simulink model "uz_typeconv_27En18_to27En15"  (R2021a)
settings: Solver=FixedStepDiscrete  StartTime=0.0  StopTime=0.1  RelTol=1e-3
values from neighbouring files (symbols this model uses):
  t_ADC = 1/f_ADC    (= 1e-05)    [uz_6ph_pu_vsd_voltages_init.m]    (also in uz_mpc_6ph_init.m; uz_mpc_6ph_state_machine_init.m; uz_typeconv_init.m)
libraries: simulink x1
settings Model: DataTypeOverride=Off  Creator=micha  LastModifiedBy=micha
settings SolverCC: AlgebraicLoopSolver=TrustRegion
settings DataIOCC: LimitDataPoints=on  SaveOutput=off  SaveTime=off
settings OptimizationCC: BlockReduction=off  ConditionallyExecuteInputs=off  DefaultParameterBehavior=Inlined  LifeSpan=inf
settings DebuggingCC: AlgebraicLoopMsg=error  SingleTaskRateTransMsg=error  AllowSymbolicDim=off  StrictBusMsg=ErrorOnBusTreatedAsVector  SFUnexpectedBacktrackingDiag=warning  SFNoUnconditionalDefaultTransitionDiag=warning  SFExecutionAtInitializationDiag=none  SFMachineParentedDataDiag=warning  ArithmeticOperatorsInVariantConditions=warning
settings HardwareCC: ProdBitPerPointer=32  ProdBitPerSizeT=32  ProdBitPerPtrDiffT=32  ProdLargestAtomicFloat=None  ProdIntDivRoundTo=Undefined  ProdEndianess=Unspecified  ProdWordSize=32  ProdHWDeviceType=ASIC/FPGA->ASIC/FPGA  ProdEqTarget=off
settings SFSimCC: SimUseLocalCustomCode=off  CustomCodeUndefinedFunction=UseInterfaceOnly
settings RTWCC: RTWUseLocalCustomCode=off
settings CodeAppCC: StateflowObjectComments=on
settings GRTTargetCC: TargetLangStandard=C89/C90 (ANSI)
settings ConfigComp: CovScope=ReferencedModels  CovMetricSettings=dw  CovSaveCumulativeToWorkspaceVar=on  CovSaveSingleToWorkspaceVar=on  CovExternalEMLEnable=off  CovSFcnEnable=off

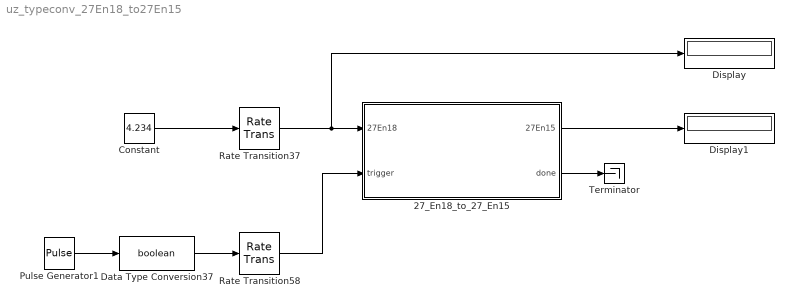
== system uz_typeconv_27En18_to27En15 ==
  27_En18_to_27_En15 : Subsystem  TreatAsAtomicUnit=on
  Constant : Constant  Value=4.234  OutDataTypeStr=fixdt(1,27,18)  SampleTime=-1
  Data Type Conversion37 : DataTypeConversion  OutDataTypeStr=boolean
  Display : Display
  Display1 : Display
  Pulse Generator1 : DiscretePulseGenerator  PulseType=Time based  Period=t_ADC  PulseWidth=5
  Rate Transition37 : RateTransition  OutPortSampleTime=t_clock
  Rate Transition58 : RateTransition  OutPortSampleTime=t_clock
  Terminator : Terminator
  wires:
  Constant/1 -> Rate Transition37/1
  27_En18_to_27_En15/1(27En15) -> Display1/1
  Data Type Conversion37/1 -> Rate Transition58/1
  Pulse Generator1/1 -> Data Type Conversion37/1
  Rate Transition58/1 -> 27_En18_to_27_En15/2(trigger)
  Rate Transition37/1 -> Display/1, 27_En18_to_27_En15/1(27En18)
  27_En18_to_27_En15/2(done) -> Terminator/1

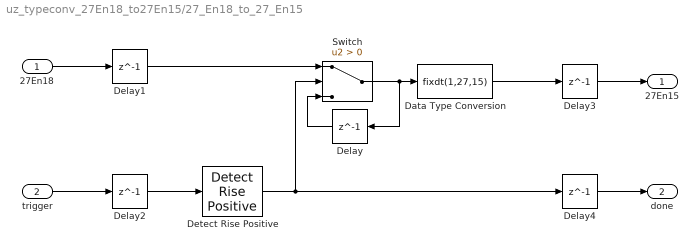
== system uz_typeconv_27En18_to27En15/27_En18_to_27_En15 ==
  27En18 : Inport
  trigger : Inport  Port=2
  Data Type Conversion : DataTypeConversion  OutDataTypeStr=fixdt(1,27,15)
  Delay{,1..4} (5 alike) : Delay  DelayLength=1
  Detect Rise Positive : simulink/Logic and Bit Operations/Detect Rise Positive  vinit=0  OutDataTypeStr=boolean
  Switch : Switch  Criteria=u2 > Threshold
  27En15 : Outport  VectorParamsAs1DForOutWhenUnconnected=off
  done : Outport  Port=2  VectorParamsAs1DForOutWhenUnconnected=off
  wires:
  Data Type Conversion/1 -> Delay3/1
  trigger/1 -> Delay2/1
  Detect Rise Positive/1 -> Switch/2, Delay4/1
  Switch/1 -> Delay/1, Data Type Conversion/1
  Delay/1 -> Switch/3
  27En18/1 -> Delay1/1
  Delay1/1 -> Switch/1
  Delay2/1 -> Detect Rise Positive/1
  Delay3/1 -> 27En15/1
  Delay4/1 -> done/1
